simulink model "SVFB_LocalObserver_notclean"  (R2023b)
settings: Solver=ode45  StartTime=0.0  StopTime=5  RelTol=1e-3
undefined symbols (not defined in the file): A, B, C, closed_loop_dynamics, closed_loop_local_observer, K0, L_luemb, S0_x0, Si_x0
settings Model: Creator=aless  LastModifiedBy=aless
settings RTWCC: GPUComputeCapability=5.0

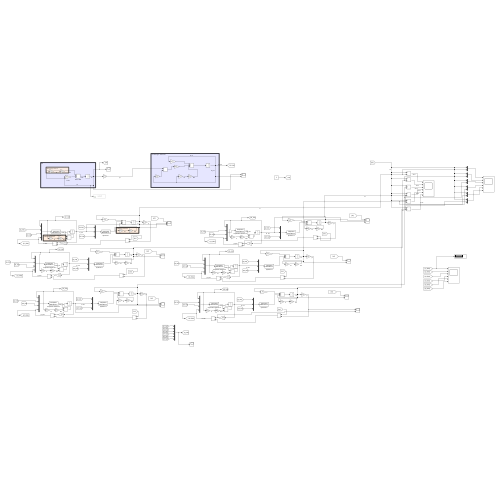
[thumbnail: Simulink's stored preview of the top-level diagram]
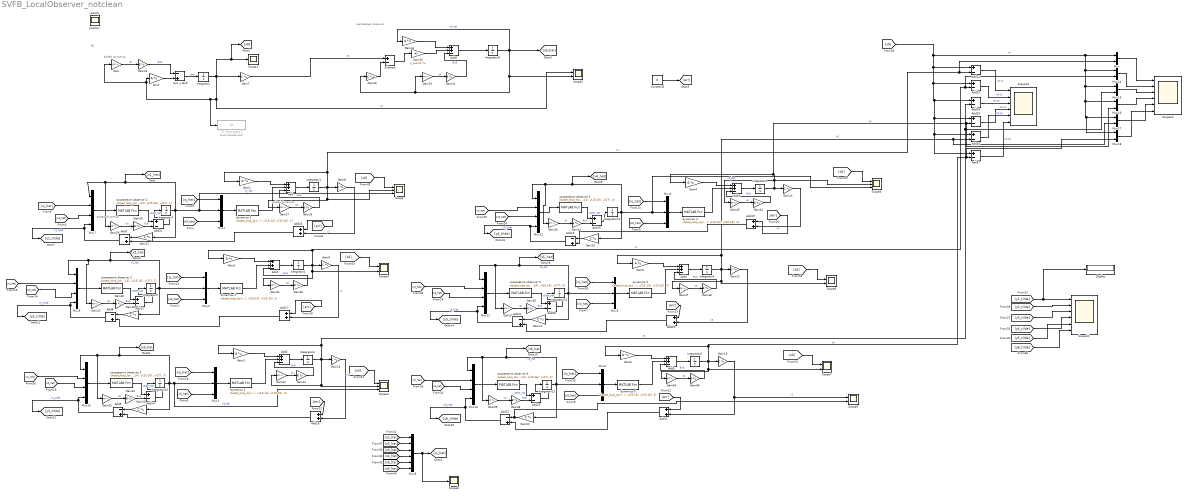
== system SVFB_LocalObserver_notclean ==
  note: added dynamics
  note: luemberger observer
  note: S0
  note: added dynamics
  note: added dynamics
  A*x0 : Gain  Gain=A  Multiplication=Matrix(K*u)
  Add{,1..6} (7 alike) : Sum  Inputs=++-
  Add{7..12} (6 alike) : Sum  Inputs=-+
  Add{13..15,22..29,31} (12 alike) : Sum  Inputs=+-
  Add{16..21} (6 alike) : Sum
  Ax0 + Bu0 : Sum  Inputs=-+
  Constant5 : Constant  Value=0
  Display : Display
  Gain{,25,27,29,31,33,35,37,39,41,43,45,47,49} (14 alike) : Gain  Gain=K0  Multiplication=Matrix(K*u)
  Gain{1..6,14} (7 alike) : Gain  Gain=A  Multiplication=Matrix(K*u)
  Gain{7..13,16..22} (14 alike) : Gain  Gain=C  Multiplication=Matrix(K*u)
  Gain15 : Gain  Gain=L_luemb  Multiplication=Matrix(K*u)
  Gain{23..24,26,28,30,32,34,36,38,40,42,44,46,48} (14 alike) : Gain  Gain=B  Multiplication=Matrix(K*u)
  Integrator : Integrator  InitialCondition=S0_x0
  Integrator{1..7,9..13} (12 alike) : Integrator  InitialCondition=Si_x0
  Integrator8 : Integrator  InitialCondition=S0_x0
  Mux{,14..18} (6 alike) : Mux  Inputs=2
  Mux{1..6} (6 alike) : Mux  Inputs=3
  Mux{7,9..13} (6 alike) : Mux
  Mux8 : Mux  Inputs=6
  Scope : Scope  NumInputPorts=3
  Scope1 : Scope
  Scope10 : Scope  NumInputPorts=6
  Scope11 : Scope  NumInputPorts=6
  Scope12 : Scope  NumInputPorts=6
  Scope{2..3,6..7,9} (5 alike) : Scope  NumInputPorts=2
  Scope4 : Scope  NumInputPorts=3
  Scope5 : Scope  NumInputPorts=3
  Scope8 : Scope
  Subtract : Sum  Inputs=+-
  To Workspace7 : ToWorkspace  Commented=on  VariableName=x0  SampleTime=-1
  cooperative observer 1 : MATLABFcn  MATLABFcn=closed_loop_local_observer(u(1:2), u(3:14), u(15:16), u(17), 1)
  cooperative observer 2 : MATLABFcn  MATLABFcn=closed_loop_local_observer(u(1:2), u(3:14), u(15:16), u(17), 2)
  cooperative observer 3 : MATLABFcn  MATLABFcn=closed_loop_local_observer(u(1:2), u(3:14), u(15:16), u(17), 3)
  cooperative observer 4 : MATLABFcn  MATLABFcn=closed_loop_local_observer(u(1:2), u(3:14), u(15:16), u(17), 4)
  cooperative observer 5 : MATLABFcn  MATLABFcn=closed_loop_local_observer(u(1:2), u(3:14), u(15:16), u(17), 5)
  cooperative observer 6 : MATLABFcn  MATLABFcn=closed_loop_local_observer(u(1:2), u(3:14), u(15:16), u(17), 6)
  dynamics 1 : MATLABFcn  MATLABFcn=closed_loop_dynamics(u(1:12), u(13:14), u(15:16), 1)
  dynamics 2 : MATLABFcn  MATLABFcn=closed_loop_dynamics(u(1:12), u(13:14), u(15:16), 2)
  dynamics 3 : MATLABFcn  MATLABFcn=closed_loop_dynamics(u(1:12), u(13:14), u(15:16), 3)
  dynamics 4 : MATLABFcn  MATLABFcn=closed_loop_dynamics(u(1:12), u(13:14), u(15:16), 4)
  dynamics 5 : MATLABFcn  MATLABFcn=closed_loop_dynamics(u(1:12), u(13:14), u(15:16), 5)
  dynamics 6 : MATLABFcn  MATLABFcn=closed_loop_dynamics(u(1:12), u(13:14), u(15:16), 6)
  position : Scope
  velocity : Scope
  wires:
  Gain21/1 -> Add11/1
  Add12/1 -> [y6_tilde], Mux13/4  "y6_tilde"
  Add7/1 -> [y1_tilde], Mux7/4  "y1_tilde"
  Gain19/1 -> Add9/1
  Gain22/1 -> Scope9/2, Add12/1
  Mux10/1 -> cooperative observer 3/1
  Add2/1 -> Integrator3/1
  Integrator10/1 -> Gain19/1, [x3_hat], Gain33/1, Mux10/1, Scope4/3, Mux3/2  "x3_hat"
  [x0_hat] -> Mux3/3
  [x0_hat] -> Mux10/3
  Mux3/1 -> dynamics 3/1
  Integrator3/1 -> Gain43/1, Scope4/2, Add24/2, Mux15/2, Gain3/1, Gain10/1  "x3"
  dynamics 3/1 -> Add2/2
  Mux11/1 -> cooperative observer 4/1
  [xj_hat] -> Mux4/1
  Mux4/1 -> dynamics 4/1
  Gain3/1 -> Add2/1
  Integrator4/1 -> Gain45/1, Scope5/2, Mux16/2, Add25/2, Gain4/1, Gain11/1  "x4"
  Add3/1 -> Integrator4/1
  Integrator11/1 -> Gain20/1, [x4_hat], Gain35/1, Mux11/1, Scope5/3, Mux4/2  "x4_hat"
  dynamics 4/1 -> Add3/2
  Gain4/1 -> Add3/1
  Mux12/1 -> cooperative observer 5/1
  [xj_hat] -> Mux5/1
  Add4/1 -> Integrator5/1
  Integrator12/1 -> Gain21/1, [x5_hat], Gain37/1, Mux12/1, Mux5/2  "x5_hat"
  [x0_hat] -> Mux12/3
  dynamics 5/1 -> Add4/2
  Integrator5/1 -> Scope6/2, Gain47/1, Mux17/2, Add26/2, Gain5/1, Gain12/1  "x5"
  [xj_hat] -> Mux12/2
  [x0_hat] -> Mux5/3
  [x5_hat] -> Mux8/5
  [x3_hat] -> Mux8/3
  [x0_hat] -> Mux11/3
  [x2_hat] -> Mux8/2
  Gain18/1 -> Add8/1
  dynamics 2/1 -> Add1/2
  Gain2/1 -> Add1/1
  Integrator2/1 -> Gain41/1, Scope3/2, Mux14/2, Add23/2, Gain2/1, Gain9/1  "x2"
  Add10/1 -> [y4_tilde], Mux11/4  "y4_tilde"
  Mux2/1 -> dynamics 2/1
  Gain5/1 -> Add4/1
  [x0_hat] -> Mux9/3
  [x0_hat] -> Mux2/3
  [xj_hat] -> Mux9/2
  Add11/1 -> [y5_tilde], Mux12/4  "y5_tilde"
  [xj_hat] -> Mux2/1
  Integrator9/1 -> Gain18/1, [x2_hat], Gain31/1, Mux9/1, Mux2/2  "x2_hat"
  Add1/1 -> Integrator2/1
  Add5/1 -> Integrator6/1
  Mux13/1 -> cooperative observer 6/1
  [x0_hat] -> Mux4/3
  Integrator13/1 -> Gain22/1, [x6_hat], Gain39/1, Mux13/1, Mux6/2  "x6_hat"
  [x0_hat] -> Mux6/3
  Mux9/1 -> cooperative observer 2/1
  Mux6/1 -> dynamics 6/1
  [xj_hat] -> Mux6/1
  Integrator6/1 -> Gain49/1, Scope7/2, Mux18/2, Add27/2, Gain6/1, Gain13/1  "x6"
  Gain20/1 -> Add10/1
  [x6_hat] -> Mux8/6
  Add8/1 -> [y2_tilde], Mux9/4  "y2_tilde"
  Add9/1 -> [y3_tilde], Mux10/4  "y3_tilde"
  Gain6/1 -> Add5/1
  Mux5/1 -> dynamics 5/1
  Mux7/1 -> cooperative observer 1/1
  [xj_hat] -> Mux7/2
  [xj_hat] -> Mux3/1
  [x0_hat] -> Mux1/3
  [xj_hat] -> Mux1/1
  Mux8/1 -> [xj_hat], Scope8/1
  [x1_hat] -> Mux8/1
  dynamics 6/1 -> Add5/2
  Integrator7/1 -> Gain17/1, [x1_hat], Gain29/1, Mux7/1, Scope/3, Mux1/2  "x1_hat"
  [xj_hat] -> Mux13/2
  [x0] -> Scope/1
  [xj_hat] -> Mux10/2
  [x0_hat] -> Mux7/3
  Integrator1/1 -> Mux/2, Add22/2, Gain1/1, Gain8/1, Gain27/1, Scope/2  "x1"
  dynamics 1/1 -> Add/2
  [x4_hat] -> Mux8/4
  Add/1 -> Integrator1/1
  [x0_hat] -> Mux13/3
  Mux1/1 -> dynamics 1/1
  Gain1/1 -> Add/1
  [xj_hat] -> Mux11/2
  [x0] -> Scope3/1
  [x0] -> Scope4/1
  [x0] -> Scope5/1
  [x0] -> Scope6/1
  [x0] -> Scope7/1
  Gain17/1 -> Add7/1
  Constant5/1 -> [err]
  Gain8/1 -> Add16/2  "y1"
  [err] -> Add16/1
  Add16/1 -> Add7/2
  Add17/1 -> Add8/2
  [err] -> Add17/1
  Gain9/1 -> Add17/2  "y2"
  Add18/1 -> Add9/2
  Gain10/1 -> Add18/2  "y3"
  [err] -> Add18/1
  [err] -> Add19/1
  Gain11/1 -> Add19/2  "y4"
  Add19/1 -> Add10/2
  [err] -> Add20/1
  Gain12/1 -> Add20/2  "y5"
  Add20/1 -> Add11/2
  Add21/1 -> Add12/2
  [err] -> Add21/1
  Gain13/1 -> Scope9/1, Add21/2  "y1"
  [x0] -> Mux18/1, Mux17/1, Mux16/1, Mux15/1, Mux14/1, Mux/1, Add22/1, Add23/1, Add24/1, Add25/1, Add26/1, Add27/1  "x0"
  [y1_tilde] -> Display/1, Scope11/1
  [y2_tilde] -> Scope11/2
  [y3_tilde] -> Scope11/3
  [y4_tilde] -> Scope11/4
  [y5_tilde] -> Scope11/5
  [y6_tilde] -> Scope11/6
  Add22/1 -> Scope10/1  "x0-x1"
  Add23/1 -> Scope10/2  "x0-x2"
  Add24/1 -> Scope10/3  "x0-x3"
  Add25/1 -> Scope10/4  "x0-x4"
  Add26/1 -> Scope10/5  "x0-x5"
  Add27/1 -> Scope10/6  "x0-x6"
  A*x0/1 -> Ax0 + Bu0/2
  Gain15/1 -> Add6/2
  Integrator8/1 -> Gain14/1, [x0_hat], Gain25/1, Gain16/1, Scope2/2  "x0_hat"
  Subtract/1 -> Gain15/1
  Add6/1 -> Integrator8/1
  Gain14/1 -> Add6/1
  Gain/1 -> Gain23/1  "u0"
  Gain25/1 -> Gain24/1  "u0"
  Ax0 + Bu0/1 -> Integrator/1  "dx0"
  Gain23/1 -> Ax0 + Bu0/1  "Bu0"
  Gain7/1 -> Subtract/1  "y0"
  Integrator/1 -> [x0], Scope1/1, Gain7/1, Scope2/1, To Workspace7/1, Gain/1, A*x0/1  "x0"
  Gain24/1 -> Add6/3  "Bu0"
  Gain16/1 -> Subtract/2
  Gain27/1 -> Gain26/1  "u0"
  Gain26/1 -> Add/3  "Bu0"
  Gain29/1 -> Gain28/1  "u0"
  Gain28/1 -> Add31/2  "Bu0"
  Add31/1 -> Integrator7/1
  cooperative observer 1/1 -> Add31/1  "x1dot_hat"
  Gain31/1 -> Gain30/1  "u0"
  Gain30/1 -> Add13/2  "Bu0"
  Add13/1 -> Integrator9/1
  cooperative observer 2/1 -> Add13/1  "x2dot_hat"
  Gain33/1 -> Gain32/1  "u0"
  Gain32/1 -> Add14/2  "Bu0"
  Add14/1 -> Integrator10/1
  cooperative observer 3/1 -> Add14/1  "x3dot_hat"
  Gain35/1 -> Gain34/1  "u0"
  Gain34/1 -> Add15/2  "Bu0"
  Add15/1 -> Integrator11/1
  cooperative observer 4/1 -> Add15/1  "x4dot_hat"
  Gain37/1 -> Gain36/1  "u0"
  Gain36/1 -> Add28/2  "Bu0"
  Add28/1 -> Integrator12/1
  cooperative observer 5/1 -> Add28/1  "x5dot_hat"
  Gain39/1 -> Gain38/1  "u0"
  Gain38/1 -> Add29/2  "Bu0"
  cooperative observer 6/1 -> Add29/1  "x6dot_hat"
  Add29/1 -> Integrator13/1
  Mux/1 -> Scope12/1
  Mux14/1 -> Scope12/2
  Mux15/1 -> Scope12/3
  Mux16/1 -> Scope12/4
  Mux17/1 -> Scope12/5
  Mux18/1 -> Scope12/6
  Gain41/1 -> Gain40/1  "u0"
  Gain40/1 -> Add1/3  "Bu0"
  Gain43/1 -> Gain42/1  "u0"
  Gain42/1 -> Add2/3  "Bu0"
  Gain45/1 -> Gain44/1  "u0"
  Gain44/1 -> Add3/3  "Bu0"
  Gain47/1 -> Gain46/1  "u0"
  Gain46/1 -> Add4/3  "Bu0"
  Gain49/1 -> Gain48/1  "u0"
  Gain48/1 -> Add5/3  "Bu0"
